simulink model "SimuMCCEchant"  (R2017b)
settings: Solver=VariableStepAuto  StartTime=0.0  StopTime=Tf  FixedStep=1e-4  MaxStep=1e-4  RelTol=1e-3
undefined symbols (not defined in the file): C0, Cl, DiscIntNeverNeededParam, F, Imax, J, Kelec, Kmeca, Kphi, L, nbpts, PWMmax, R, R20, R22, R23, Rshunt, Ts, Tsmeca, Vcc, Vdc
libraries: simulink_extras x1
settings Model: Creator=romaindelpoux  LastModifiedBy=Lubin Kerhuel
settings SolverCC: ZeroCrossControl=DisableAll

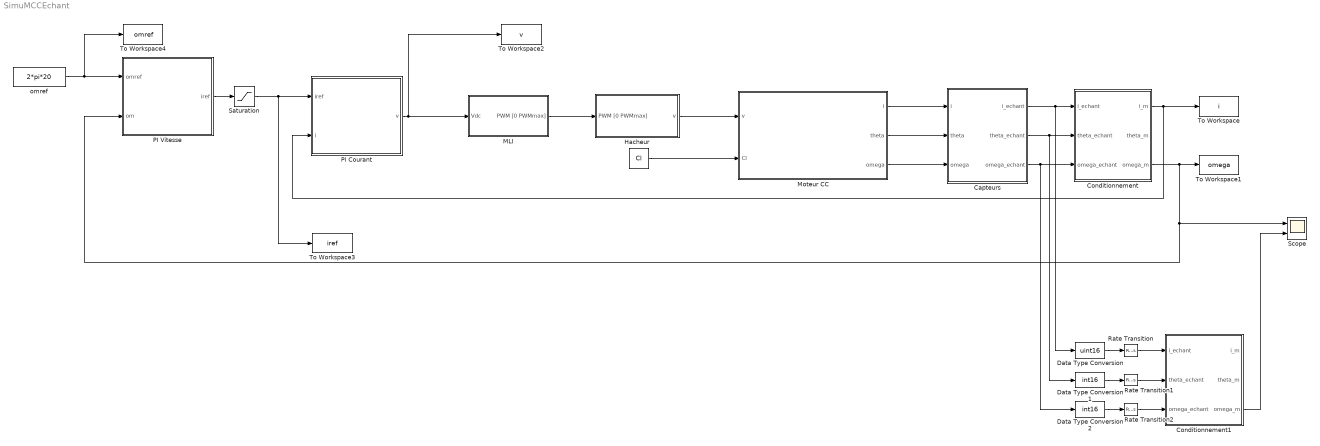
== system SimuMCCEchant ==
  " " : Constant  Value=Cl
  Capteurs : Subsystem
  Conditionnement : Subsystem
  Conditionnement1 : Subsystem
  Data Type Conversion : DataTypeConversion  OutDataTypeStr=uint16
  Data Type Conversion1 : DataTypeConversion  OutDataTypeStr=int16
  Data Type Conversion2 : DataTypeConversion  OutDataTypeStr=int16
  Hacheur : Subsystem
  MLI : Subsystem
  Moteur CC : Subsystem
  PI Courant : Subsystem  TreatAsAtomicUnit=on
  "PI Vitesse " : Subsystem  TreatAsAtomicUnit=on
  Rate Transition : RateTransition  Deterministic=off  OutPortSampleTime=Ts
  Rate Transition1 : RateTransition  Deterministic=off  OutPortSampleTime=Ts
  Rate Transition2 : RateTransition  Deterministic=off  OutPortSampleTime=Ts
  Saturation : Saturate  UpperLimit=Imax  LowerLimit=-Imax
  Scope : Scope  NumInputPorts=2
  To Workspace : ToWorkspace  VariableName=i  SaveFormat=Timeseries  SampleTime=-1
  To Workspace1 : ToWorkspace  VariableName=omega  SaveFormat=Timeseries  SampleTime=-1
  To Workspace2 : ToWorkspace  VariableName=v  SaveFormat=Timeseries  SampleTime=-1
  To Workspace3 : ToWorkspace  VariableName=iref  SaveFormat=Timeseries  SampleTime=-1
  To Workspace4 : ToWorkspace  VariableName=omref  SaveFormat=Timeseries  SampleTime=-1
  omref : Constant  Value=2*pi*20
  wires:
  omref/1 -> "PI Vitesse "/1(omref), To Workspace4/1
  " "/1 -> Moteur CC/2(Cl)
  "PI Vitesse "/1(iref) -> Saturation/1
  Moteur CC/1(i) -> Capteurs/1(i)
  Moteur CC/2(theta) -> Capteurs/2(theta)
  Capteurs/1(i_echant) -> Data Type Conversion/1, Conditionnement/1(i_echant)
  Capteurs/2(theta_echant) -> Data Type Conversion1/1, Conditionnement/2(theta_echant)
  Conditionnement/1(i_m) -> PI Courant/2(i), To Workspace/1
  Conditionnement/3(omega_m) -> To Workspace1/1, "PI Vitesse "/2(om), Scope/1
  PI Courant/1(v) -> MLI/1(Vdc), To Workspace2/1
  Moteur CC/3(omega) -> Capteurs/3(omega)
  Capteurs/3(omega_echant) -> Data Type Conversion2/1, Conditionnement/3(omega_echant)
  Saturation/1 -> PI Courant/1(iref), To Workspace3/1
  MLI/1(PWM [0 PWMmax]) -> Hacheur/1(PWM [0 PWMmax])
  Hacheur/1(v) -> Moteur CC/1(v)
  Rate Transition/1 -> Conditionnement1/1(i_echant)
  Rate Transition1/1 -> Conditionnement1/2(theta_echant)
  Rate Transition2/1 -> Conditionnement1/3(omega_echant)
  Data Type Conversion/1 -> Rate Transition/1
  Data Type Conversion1/1 -> Rate Transition1/1
  Data Type Conversion2/1 -> Rate Transition2/1
  Conditionnement1/3(omega_m) -> Scope/2

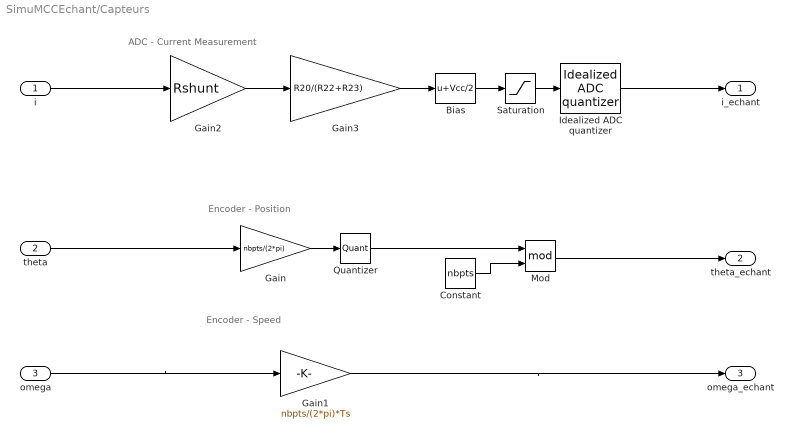
== system SimuMCCEchant/Capteurs ==
  note: ADC - Current Measurement
  note: Encoder - Speed
  note: Encoder - Position
  i : Inport
  theta : Inport  Port=2
  omega : Inport  Port=3
  Bias : Bias  Bias=Vcc/2
  Constant : Constant  Value=nbpts
  Gain : Gain  Gain=nbpts/(2*pi)
  Gain1 : Gain  Gain=nbpts/(2*pi)*Ts
  Gain2 : Gain  Gain=Rshunt
  Gain3 : Gain  Gain=R20/(R22+R23)
  Idealized ADC quantizer : simulink_extras/Additional Discrete/Idealized ADC quantizer  NumberOfConverterBits=10  Vmin=0  Vmax=Vcc  OutputDataType=double  OutputNegativeValues=off
      settings: SourceProductName=Simulink
  Mod : Math  Operator=mod  SaturateOnIntegerOverflow=on
  Quantizer : Quantizer  QuantizationInterval=1
  Saturation : Saturate  UpperLimit=Vcc  LowerLimit=0
  i_echant : Outport
  theta_echant : Outport  Port=2
  omega_echant : Outport  Port=3
  wires:
  theta/1 -> Gain/1
  i/1 -> Gain2/1
  Gain3/1 -> Bias/1
  Gain/1 -> Quantizer/1
  Gain2/1 -> Gain3/1
  Saturation/1 -> Idealized ADC quantizer/1
  Bias/1 -> Saturation/1
  Idealized ADC quantizer/1 -> i_echant/1
  Quantizer/1 -> Mod/1
  Gain1/1 -> omega_echant/1
  omega/1 -> Gain1/1
  Constant/1 -> Mod/2
  Mod/1 -> theta_echant/1

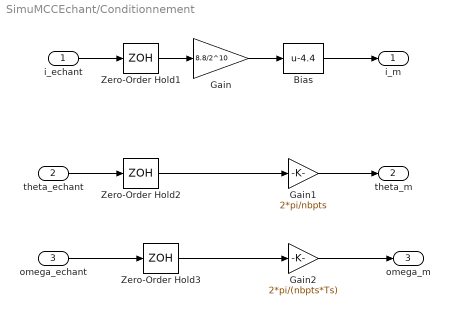
== system SimuMCCEchant/Conditionnement ==
  i_echant : Inport
  theta_echant : Inport  Port=2
  omega_echant : Inport  Port=3
  Bias : Bias  Bias=-4.4
  Gain : Gain  Gain=8.8/2^10
  Gain1 : Gain  Gain=2*pi/nbpts
  Gain2 : Gain  Gain=2*pi/(nbpts*Ts)
  Zero-Order Hold1 : ZeroOrderHold  SampleTime=Ts
  Zero-Order Hold2 : ZeroOrderHold  SampleTime=Ts
  Zero-Order Hold3 : ZeroOrderHold  SampleTime=Ts
  i_m : Outport
  theta_m : Outport  Port=2
  omega_m : Outport  Port=3
  wires:
  Gain1/1 -> theta_m/1
  i_echant/1 -> Zero-Order Hold1/1
  Gain/1 -> Bias/1
  Bias/1 -> i_m/1
  theta_echant/1 -> Zero-Order Hold2/1
  Zero-Order Hold1/1 -> Gain/1
  Zero-Order Hold2/1 -> Gain1/1
  Zero-Order Hold3/1 -> Gain2/1
  Gain2/1 -> omega_m/1
  omega_echant/1 -> Zero-Order Hold3/1

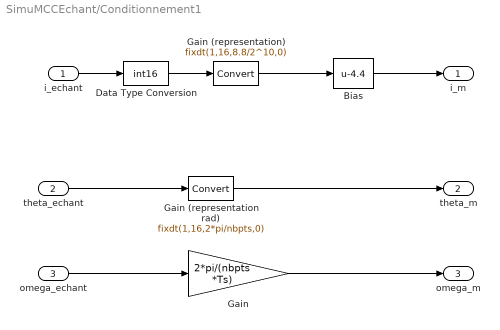
== system SimuMCCEchant/Conditionnement1 ==
  i_echant : Inport
  theta_echant : Inport  Port=2
  omega_echant : Inport  Port=3
  Bias : Bias  Bias=-4.4
  Data Type Conversion : DataTypeConversion  OutDataTypeStr=int16
  Gain : Gain  Gain=2*pi/(nbpts *Ts)  OutMin=[-100]  OutMax=[100]  OutDataTypeStr=fixdt(1,16)
  Gain (representation rad) : DataTypeConversion  OutDataTypeStr=fixdt(1,16,2*pi/nbpts,0)  ConvertRealWorld=Stored Integer (SI)
  Gain (representation) : DataTypeConversion  OutDataTypeStr=fixdt(1,16,8.8/2^10,0)  ConvertRealWorld=Stored Integer (SI)
  i_m : Outport
  theta_m : Outport  Port=2
  omega_m : Outport  Port=3
  wires:
  Gain/1 -> omega_m/1
  omega_echant/1 -> Gain/1
  theta_echant/1 -> Gain (representation rad)/1
  i_echant/1 -> Data Type Conversion/1
  Bias/1 -> i_m/1
  Gain (representation)/1 -> Bias/1
  Gain (representation rad)/1 -> theta_m/1
  Data Type Conversion/1 -> Gain (representation)/1

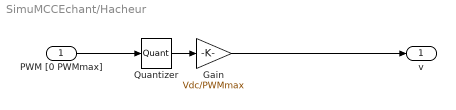
== system SimuMCCEchant/Hacheur ==
  PWM [0 PWMmax] : Inport
  Gain : Gain  Gain=Vdc/PWMmax
  Quantizer : Quantizer  QuantizationInterval=1
  v : Outport
  wires:
  PWM [0 PWMmax]/1 -> Quantizer/1
  Quantizer/1 -> Gain/1
  Gain/1 -> v/1

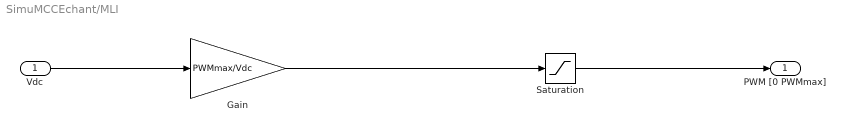
== system SimuMCCEchant/MLI ==
  Vdc : Inport
  Gain : Gain  Gain=PWMmax/Vdc
  Saturation : Saturate  UpperLimit=PWMmax
  PWM [0 PWMmax] : Outport
  wires:
  Vdc/1 -> Gain/1
  Gain/1 -> Saturation/1
  Saturation/1 -> PWM [0 PWMmax]/1

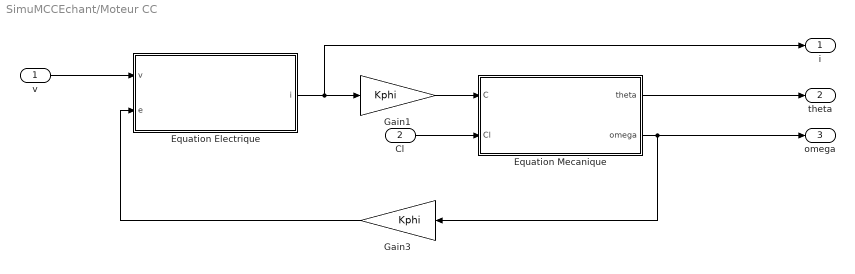
== system SimuMCCEchant/Moteur CC ==
  v : Inport
  Cl : Inport  Port=2
  Equation Electrique : Subsystem
  Equation Mecanique : Subsystem
  Gain1 : Gain  Gain=Kphi
  "Gain3  " : Gain  Gain=Kphi
  i : Outport
  theta : Outport  Port=2
  omega : Outport  Port=3
  wires:
  "Gain3  "/1 -> Equation Electrique/2(e)
  Gain1/1 -> Equation Mecanique/1(C)
  Cl/1 -> Equation Mecanique/2(Cl)
  v/1 -> Equation Electrique/1(v)
  Equation Electrique/1(i) -> i/1, Gain1/1
  Equation Mecanique/2(omega) -> "Gain3  "/1, omega/1
  Equation Mecanique/1(theta) -> theta/1

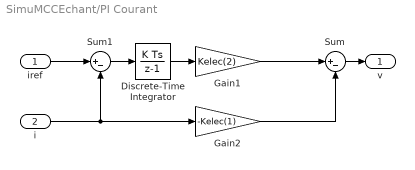
== system SimuMCCEchant/PI Courant ==
  iref : Inport
  i : Inport  Port=2
  Discrete-Time Integrator : DiscreteIntegrator  InitialConditionSetting=State (most efficient)  SampleTime=-1  ICPrevOutput=DiscIntNeverNeededParam  ICPrevScaledInput=DiscIntNeverNeededParam
  Gain1 : Gain  Gain=Kelec(2)
  Gain2 : Gain  Gain=-Kelec(1)
  Sum : Sum  Inputs=|+-
  Sum1 : Sum  Inputs=|+-
  v : Outport
  wires:
  iref/1 -> Sum1/1
  i/1 -> Gain2/1, Sum1/2
  Sum1/1 -> Discrete-Time Integrator/1
  Discrete-Time Integrator/1 -> Gain1/1
  Sum/1 -> v/1
  Gain1/1 -> Sum/1
  Gain2/1 -> Sum/2

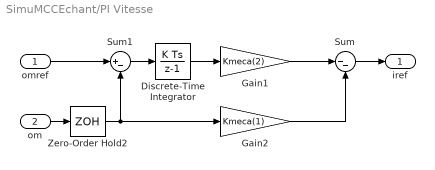
== system SimuMCCEchant/PI Vitesse  ==
  omref : Inport
  om : Inport  Port=2
  Discrete-Time Integrator : DiscreteIntegrator  InitialConditionSetting=State (most efficient)  SampleTime=-1  ICPrevOutput=DiscIntNeverNeededParam  ICPrevScaledInput=DiscIntNeverNeededParam
  Gain1 : Gain  Gain=Kmeca(2)
  Gain2 : Gain  Gain=Kmeca(1)
  Sum : Sum  Inputs=|--
  Sum1 : Sum  Inputs=|+-
  Zero-Order Hold2 : ZeroOrderHold  SampleTime=Tsmeca
  iref : Outport
  wires:
  omref/1 -> Sum1/1
  om/1 -> Zero-Order Hold2/1
  Sum1/1 -> Discrete-Time Integrator/1
  Discrete-Time Integrator/1 -> Gain1/1
  Sum/1 -> iref/1
  Gain1/1 -> Sum/1
  Gain2/1 -> Sum/2
  Zero-Order Hold2/1 -> Sum1/2, Gain2/1

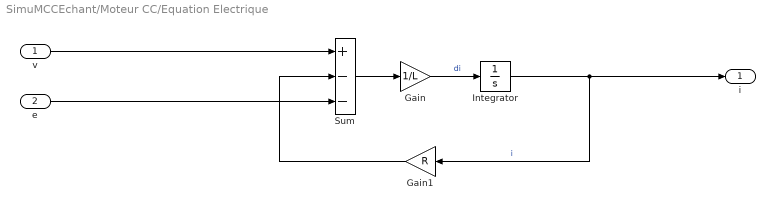
== system SimuMCCEchant/Moteur CC/Equation Electrique ==
  v : Inport
  e : Inport  Port=2
  Gain : Gain  Gain=1/L
  Gain1 : Gain  Gain=R
  Integrator : Integrator
  Sum : Sum  Inputs=+--
  i : Outport
  wires:
  Gain1/1 -> Sum/2
  Sum/1 -> Gain/1
  Integrator/1 -> i/1, Gain1/1  "i"
  Gain/1 -> Integrator/1  "di"
  v/1 -> Sum/1
  e/1 -> Sum/3

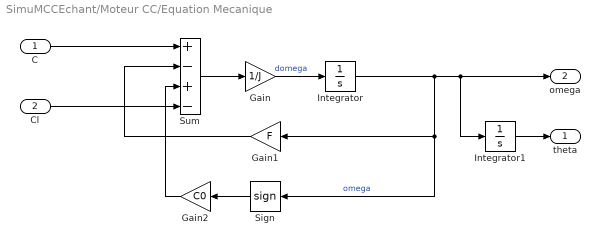
== system SimuMCCEchant/Moteur CC/Equation Mecanique ==
  C : Inport
  Cl : Inport  Port=2
  Gain : Gain  Gain=1/J
  Gain1 : Gain  Gain=F
  Gain2 : Gain  Gain=C0
  Integrator : Integrator
  Integrator1 : Integrator
  Sign : Signum
  Sum : Sum  Inputs=+-+-
  theta : Outport
  omega : Outport  Port=2
  wires:
  Gain/1 -> Integrator/1  "domega"
  Integrator/1 -> Sign/1, Gain1/1, Integrator1/1, omega/1  "omega"
  Sum/1 -> Gain/1
  Gain1/1 -> Sum/2
  Sign/1 -> Gain2/1
  Gain2/1 -> Sum/3
  C/1 -> Sum/1
  Cl/1 -> Sum/4
  Integrator1/1 -> theta/1
